simulink model "TrajectoryFunctionForModel"  (R2020b)
settings: Solver=VariableStepAuto  StartTime=0.0  StopTime=10.0  RelTol=1e-3
values from neighbouring files (symbols this model uses):
  theta = 60    [ProjectileModelParameter.m]
  v0 = 35    [ProjectileModelParameter.m]
  x0 = -35    [ProjectileModelParameter.m]
  y0 = 0    [ProjectileModelParameter.m]
libraries: simulink x1
settings Model: Creator=user  LastModifiedBy=user

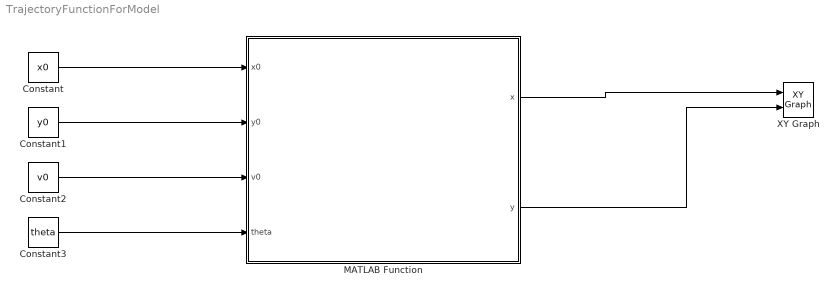
== system TrajectoryFunctionForModel ==
  Constant : Constant  Value=x0
  Constant1 : Constant  Value=y0
  Constant2 : Constant  Value=v0
  Constant3 : Constant  Value=theta
  MATLAB Function : MATLAB Function  TreatAsAtomicUnit=on
  XY Graph : simulink/Sinks/XY Graph  xmin=0  xmax=1000  ymin=0  ymax=1000  st=1
  wires:
  Constant/1 -> MATLAB Function/1(x0)
  Constant1/1 -> MATLAB Function/2(y0)
  Constant2/1 -> MATLAB Function/3(v0)
  Constant3/1 -> MATLAB Function/4(theta)
  MATLAB Function/1(x) -> XY Graph/1
  MATLAB Function/2(y) -> XY Graph/2

== matlab function TrajectoryFunctionForModel/MATLAB Function ==
  data: x output; x0 input; y output; y0 input; v0 input; theta input
function [x,y] = TrajectoryFunction(x0,y0,v0,theta)
g=9.81;
vx=v0*cos(theta);
vy=v0*sin(theta);
tf=2*vy/g;
t=linspace(0,tf,30);
 %x and y Equations
x=x0+vx*t;
y=y0+vy*t-(g*t.^2)/2;
%Maximum Height
%hmax=(v0^2*sin(theta)^2)/(2*g);
end
